simulink model "x25_CPM_130_Causal_BO_Courant"  (R2024b)
settings: Solver=VariableStepAuto  StartTime=0.0  StopTime=0.84  RelTol=1e-3
InitFcn:
  | run("parametres.m")
  | %data = lire_csv_rc4("Echelon_CH_P50_HG.csv")
values from neighbouring files (symbols this model uses):
  fv = 2.78e-6    (= 2.78e-06)    [parametres.m]
  Jm = 2e-6    (= 2e-06)    [parametres.m]
  Kcapt = 512*4/2/pi    (= 325.949323452)    [parametres.m]
  Kcm = 25.6e-3    (= 0.0256)    [parametres.m]
  KCou_I = 270    [parametres.m]
  KCou_P = 670    [parametres.m]
  Kem = 1/(373 *2*pi/60)    (= 0.0256013313285)    [parametres.m]
  Lm = 0.278e-3    (= 0.000278)    [parametres.m]
  pas = 5 /2/pi    (= 0.795774715459)    [parametres.m]
  r = 1/16    (= 0.0625)    [parametres.m]
  Rm = 2.15    [parametres.m]
  USAT = 24    [parametres.m]
undefined symbols (not defined in the file or in its folder): Cfs
settings Model: Creator=xavier.pessoles2  LastModifiedBy=xpess

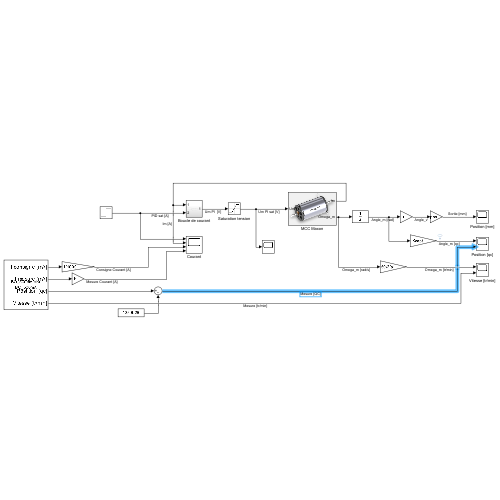
[thumbnail: Simulink's stored preview of the top-level diagram]
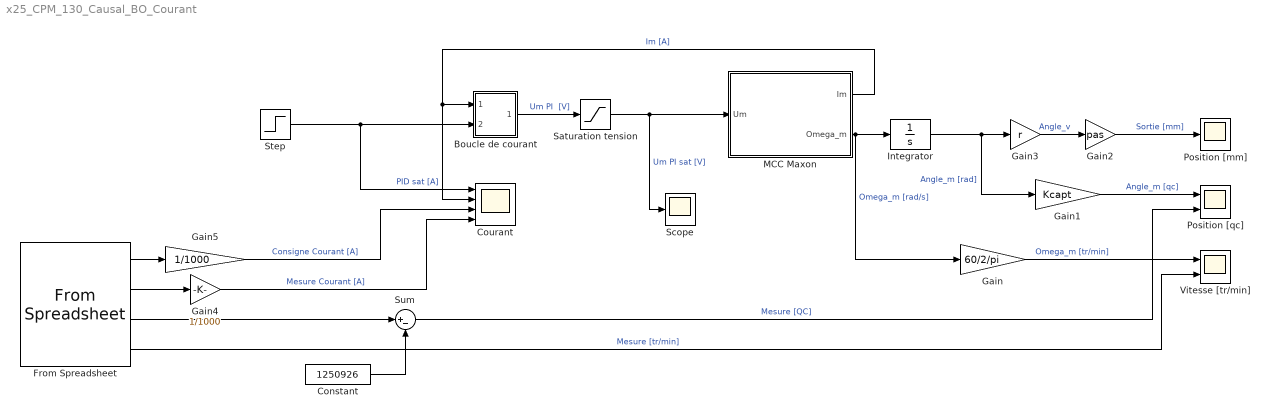
== system x25_CPM_130_Causal_BO_Courant ==
  Boucle de courant : Subsystem
  Constant : Constant  Value=1250926
  Courant : Scope  NumInputPorts=4
  From Spreadsheet : FromSpreadsheet  FileName=BO_500mA.xlsx  SheetName=BO_500mA
  Gain : Gain  Gain=60/2/pi
  Gain1 : Gain  Gain=Kcapt
  Gain2 : Gain  Gain=pas
  Gain3 : Gain  Gain=r
  Gain4 : Gain  Gain=1/1000
  Gain5 : Gain  Gain=1/1000
  Integrator : Integrator
  MCC Maxon : Subsystem
      mask Display: image('MCC.png');
  Position [mm] : Scope
  Position [qc] : Scope  NumInputPorts=2
  Saturation tension : Saturate  UpperLimit=USAT  LowerLimit=-USAT
  Scope : Scope
  Step : Step  Time=0.069  After=.5  SampleTime=0
  Sum : Sum  Inputs=|+-
  Vitesse [tr/min] : Scope  NumInputPorts=2
  wires:
  MCC Maxon/2(Omega_m) -> Gain/1, Integrator/1  "Omega_m [rad/s]"
  MCC Maxon/1(Im) -> Boucle de courant/1(In1), Courant/2  "Im [A]"
  Boucle de courant/1(Out1) -> Saturation tension/1  "Um PI  [V]"
  Gain2/1 -> Position [mm]/1  "Sortie [mm]"
  Saturation tension/1 -> Scope/1, MCC Maxon/1(Um)  "Um PI sat [V]"
  Step/1 -> Courant/1, Boucle de courant/2(In2)  "PID sat [A]"
  Integrator/1 -> Gain1/1, Gain3/1  "Angle_m [rad]"
  Gain3/1 -> Gain2/1  "Angle_v"
  Gain/1 -> Vitesse [tr/min]/1  "Omega_m [tr/min]"
  Gain1/1 -> Position [qc]/1  "Angle_m [qc]"
  From Spreadsheet/2 -> Gain4/1
  From Spreadsheet/4 -> Vitesse [tr/min]/2  "Mesure [tr/min]"
  From Spreadsheet/3 -> Sum/1
  Sum/1 -> Position [qc]/2  "Mesure [QC]"
  Constant/1 -> Sum/2
  From Spreadsheet/1 -> Gain5/1
  Gain4/1 -> Courant/4  "Mesure Courant [A]"
  Gain5/1 -> Courant/3  "Consigne Courant [A]"

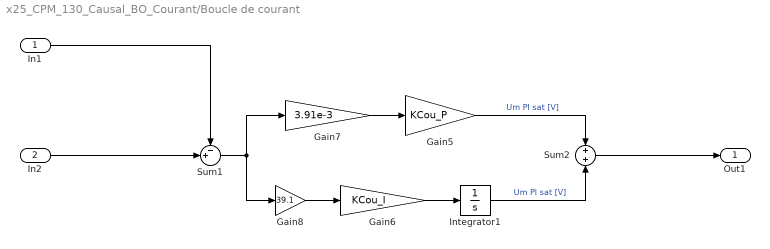
== system x25_CPM_130_Causal_BO_Courant/Boucle de courant ==
  In1 : Inport
  In2 : Inport  Port=2
  Gain5 : Gain  Gain=KCou_P
  Gain6 : Gain  Gain=KCou_I
  Gain7 : Gain  Gain=3.91e-3
  Gain8 : Gain  Gain=39.1
  Integrator1 : Integrator
  Sum1 : Sum  Inputs=-+|
  Sum2 : Sum  Inputs=+|+
  Out1 : Outport
  wires:
  Sum1/1 -> Gain7/1, Gain8/1
  Sum2/1 -> Out1/1
  Gain8/1 -> Gain6/1
  In1/1 -> Sum1/1
  Gain7/1 -> Gain5/1
  Gain6/1 -> Integrator1/1
  In2/1 -> Sum1/2
  Gain5/1 -> Sum2/1  "Um PI sat [V]"
  Integrator1/1 -> Sum2/2  "Um PI sat [V]"

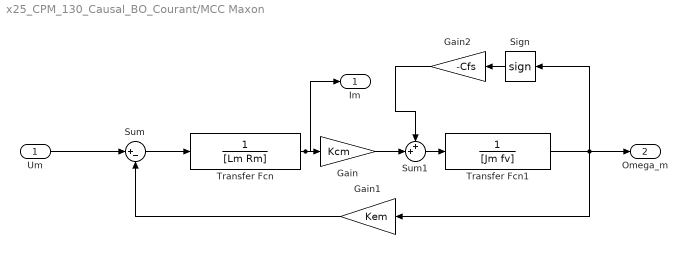
== system x25_CPM_130_Causal_BO_Courant/MCC Maxon ==
  Um : Inport
  Gain : Gain  Gain=Kcm
  Gain1 : Gain  Gain=Kem
  Gain2 : Gain  Gain=-Cfs
  Sign : Signum  ZeroCross=off
  Sum : Sum  Inputs=|+-
  Sum1 : Sum  Inputs=++|
  Transfer Fcn : TransferFcn  Denominator=[Lm Rm]
  Transfer Fcn1 : TransferFcn  Denominator=[Jm fv]
  Im : Outport
  Omega_m : Outport  Port=2
  wires:
  Transfer Fcn/1 -> Im/1, Gain/1
  Transfer Fcn1/1 -> Sign/1, Omega_m/1, Gain1/1
  Gain1/1 -> Sum/2
  Um/1 -> Sum/1
  Sum/1 -> Transfer Fcn/1
  Gain/1 -> Sum1/2
  Sum1/1 -> Transfer Fcn1/1
  Sign/1 -> Gain2/1
  Gain2/1 -> Sum1/1
